simulink model "SimulinkQ20_controle"  (R2016a)
settings: Solver=VariableStepAuto  StartTime=0.0  StopTime=10.0  RelTol=1e-3
libraries: simulink x1
settings Model: Creator=Lenovo  LastModifiedBy=Lenovo

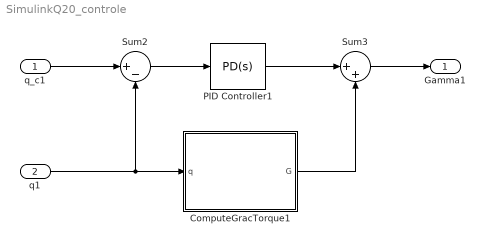
== system SimulinkQ20_controle ==
  q_c1 : Inport
  q1 : Inport  Port=2
  ComputeGracTorque1 : MATLAB Function  TreatAsAtomicUnit=on
  PID Controller1 : simulink/Continuous/PID Controller  Controller=PD  TimeDomain=Continuous-time  SampleTime=-1  IntegratorMethod=Forward Euler  FilterMethod=Forward Euler  Form=Parallel  UseFilter=on  ControllerParametersSource=internal  P=1  I=1  D=0.5  N=100  InitialConditionSource=internal  InitialConditionForIntegrator=0  InitialConditionForFilter=0  ExternalReset=none  LimitOutput=off  UpperSaturationLimit=inf  LowerSaturationLimit=-inf  LinearizeAsGain=on  AntiWindupMode=none  Kb=1  TrackingMode=off  Kt=1  PParamMin=[]  PParamMax=[]  IParamMin=[]  IParamMax=[]  DParamMin=[]  DParamMax=[]  NParamMin=[]  NParamMax=[]  KbParamMin=[]  KbParamMax=[]  KtParamMin=[]  KtParamMax=[]  POutMin=[]  POutMax=[]  IOutMin=[]  IOutMax=[]  DOutMin=[]  DOutMax=[]  NOutMin=[]  NOutMax=[]  KbOutMin=[]  KbOutMax=[]  KtOutMin=[]  KtOutMax=[]  IntegratorOutMin=[]  IntegratorOutMax=[]  FilterOutMin=[]  FilterOutMax=[]  SumOutMin=[]  SumOutMax=[]  SumI1OutMin=[]  SumI1OutMax=[]  SumI2OutMin=[]  SumI2OutMax=[]  SumI3OutMin=[]  SumI3OutMax=[]  SumDOutMin=[]  SumDOutMax=[]  SaturationOutMin=[]  SaturationOutMax=[]  IntegratorContinuousStateAttributes=''  IntegratorStateMustResolveToSignalObject=off  IntegratorRTWStateStorageClass=Auto  FilterContinuousStateAttributes=''  FilterStateMustResolveToSignalObject=off  FilterRTWStateStorageClass=Auto  DifferentiatorICPrevScaledInput=0  DifferentiatorOutMin=[]  DifferentiatorOutMax=[]
  Sum2 : Sum  Inputs=|+-
  Sum3 : Sum  Inputs=|++
  Gamma1 : Outport
  wires:
  q1/1 -> Sum2/2, ComputeGracTorque1/1(q)
  q_c1/1 -> Sum2/1
  Sum2/1 -> PID Controller1/1
  PID Controller1/1 -> Sum3/1
  ComputeGracTorque1/1(G) -> Sum3/2
  Sum3/1 -> Gamma1/1

== matlab function SimulinkQ20_controle/ComputeGracTorque1 ==
  data: q input; G output
function G = ComputeGravTorque(q)

    %Parameters
    m=[15 10 1 7 1 0.5];
    x_G1 = 0; y_G1 = 0; z_G1 = -0.25;
    x_G2 = 0.35; y_G2 = 0; z_G2 = 0;
    x_G3 = 0; y_G3 = -0.1; z_G3 = 0;
    x_G4 = 0; y_G4 = 0; z_G4 = 0;
    x_G5 = 0; y_G5 = 0; z_G5 = 0;
    x_G6 = 0; y_G6 = 0; z_G6 = 0;
    x_G = [x_G1 x_G2 x_G3 x_G4 x_G5 x_G6];
    y_G = [y_G1 y_G2 y_G3 y_G4 y_G5 y_G6];
    z_G = [z_G1 z_G2 z_G3 z_G4 z_G5 z_G6];

    d = [0 0 0.7 0 0 0];
    r = [0.5 0 0 0.2 0 0];
    alpha = [0 pi/2 0 pi/2 -pi/2 pi/2];
    theta = [q(1) q(2) q(3)+pi/2 q(4) q(5) q(6)];

    % Calculation of the Jacobian matrices of each body
    [OJv_Gi, ~] = ComputeJacGi(alpha, d, theta, r, x_G, y_G, z_G);

    %Gravity vector expressed in R0
    g = [0 0 -9.81]';

    %Calculation of the torque of gravity produced by bodies
    G = zeros(length(theta), 1);
    
    for i = 1:length(m)
        G = G - OJv_Gi(:,:,i)'*m(i)*g;
    end
end
